simulink subsystem "HallSensor"  (R2023a)
settings: Solver=VariableStepAuto  StartTime=0.0  StopTime=10.0  RelTol=1e-3
settings Model: Creator=mrrom  LastModifiedBy=mrrom

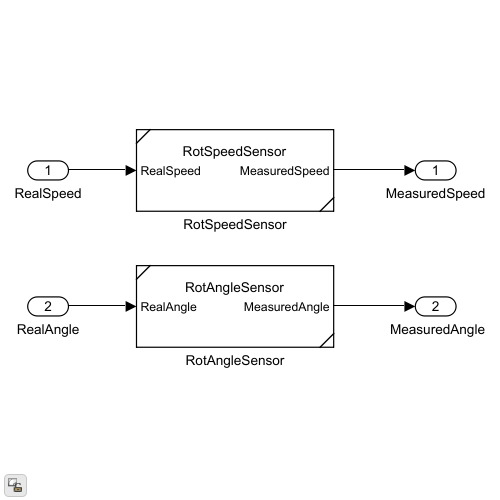
[thumbnail: Simulink's stored preview of the top-level diagram]
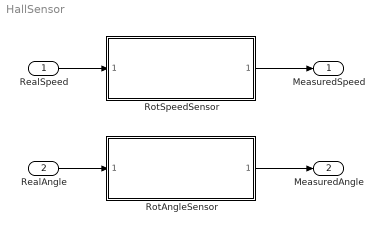
== system HallSensor ==
  RealSpeed : Inport
  RealAngle : Inport  Port=2
  RotAngleSensor : Subsystem  ReferencedSubsystem=RotAngleSensor
  RotSpeedSensor : Subsystem  ReferencedSubsystem=RotSpeedSensor
  MeasuredSpeed : Outport
  " MeasuredAngle" : Outport  Port=2
  wires:
  RealAngle/1 -> RotAngleSensor/1
  RotAngleSensor/1 -> " MeasuredAngle"/1
  RealSpeed/1 -> RotSpeedSensor/1
  RotSpeedSensor/1 -> MeasuredSpeed/1
